simulink model "bicycle_model_int"  (R2022a)
settings: Solver=FixedStepAuto  StartTime=0.0  StopTime=t_end  FixedStep=0.1  RelTol=1e-3
InitFcn:
  | bicycle_model_data
values from neighbouring files (symbols this model uses):
  b = 0.8    [TestModelv1_init.m]    (also in bicycle_model_data.m)
  D = m*a*h    (= 19.32)    [TestModelv1_init.m]    (also in bicycle_model_data.m)
  delay = 3    [TestModelv1_init.m]    (also in bicycle_model_data.m)
  g = 9.8    [TestModelv1_init.m]    (also in bicycle_model_data.m)
  h = 0.7    [TestModelv1_init.m]    (also in bicycle_model_data.m)
  hr = 0.7    [TestModelv1_init.m]    (also in bicycle_model_data.m)
  J = m*h^2    (= 45.08)    [TestModelv1_init.m]    (also in bicycle_model_data.m)
  Jr = mr*h^2    (= 36.75)    [TestModelv1_init.m]    (also in bicycle_model_data.m)
  k1 = b^2/(V^2*sin(lambda)-b*g*cos(lambda))/(m*a*c*sin(lambda))    [TestModelv1_init.m]    (also in bicycle_model_data.m)
  k2 = (b*g)/(V^2*sin(lambda)-b*g*cos(lambda))    [TestModelv1_init.m]    (also in bicycle_model_data.m = b*g/(V^2*sin(lambda)-b*g*cos(lambda)))
  m = m_rider + m_bicycle + m_otherParts    (= 92)    [TestModelv1_init.m]    (also in bicycle_model_data.m)
  mr = m_rider    (= 75)    [TestModelv1_init.m]    (also in bicycle_model_data.m)
  phi0 = 5*pi/180    (= 0.0872664625997)    [TestModelv1_init.m]    (also in bicycle_model_data.m)
  V = V_values(i)    [TestModelv1_init.m]    (also in bicycle_model_data.m = 5)
settings Model: Creator=ashut  LastModifiedBy=ashut

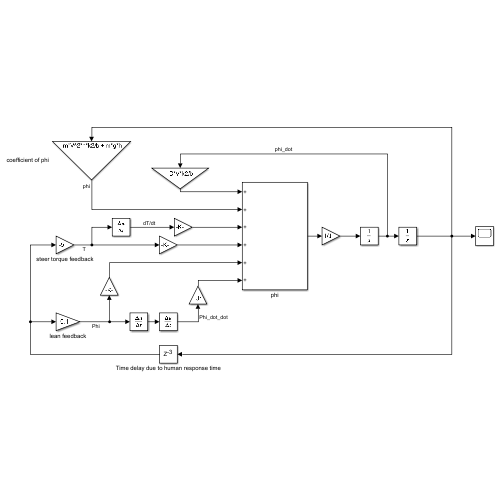
[thumbnail: Simulink's stored preview of the top-level diagram]
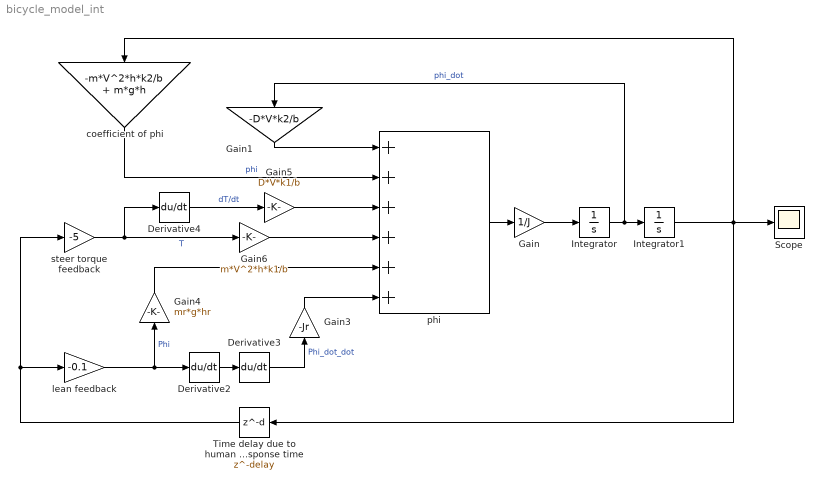
== system bicycle_model_int ==
  Derivative2 : Derivative
  Derivative3 : Derivative
  Derivative4 : Derivative
  Gain : Gain  Gain=1/J
  Gain1 : Gain  Gain=-D*V*k2/b
  Gain3 : Gain  Gain=-Jr
  Gain4 : Gain  Gain=mr*g*hr
  Gain5 : Gain  Gain=D*V*k1/b
  Gain6 : Gain  Gain=m*V^2*h*k1/b
  Integrator : Integrator
  Integrator1 : Integrator  InitialCondition=phi0
  Scope : Scope
  Time delay due to human response time : Delay  DelayLength=delay  InitialCondition=phi0
  coefficient of phi : Gain  Gain=-m*V^2*h*k2/b + m*g*h
  lean feedback : Gain  Gain=-0.1
  phi : Sum  Inputs=++++++
  steer torque feedback : Gain  Gain=-5
  wires:
  Integrator/1 -> Gain1/1, Integrator1/1  "phi_dot"
  Derivative2/1 -> Derivative3/1
  lean feedback/1 -> Derivative2/1, Gain4/1  "Phi"
  Derivative4/1 -> Gain5/1  "dT/dt"
  Gain5/1 -> phi/3
  Gain6/1 -> phi/4
  Derivative3/1 -> Gain3/1  "Phi_dot_dot"
  Gain4/1 -> phi/5
  steer torque feedback/1 -> Gain6/1, Derivative4/1  "T"
  Gain3/1 -> phi/6
  Integrator1/1 -> Time delay due to human response time/1, Scope/1, coefficient of phi/1
  Gain1/1 -> phi/1
  phi/1 -> Gain/1
  coefficient of phi/1 -> phi/2  "phi"
  Gain/1 -> Integrator/1
  Time delay due to human response time/1 -> lean feedback/1, steer torque feedback/1
